simulink model "Sim_2025_04_07_Heet"  (R2024b)
settings: Solver=FixedStepAuto  StartTime=0.0  StopTime=2350  FixedStep=0.01  RelTol=1e-3
values from neighbouring files (symbols this model uses):
  cpSn = 230    [Sim_Parameter_Heet.m]
  mB = VB*rohSn    (= 7671.14496)    [Sim_Parameter_Heet.m]
  TU = 35    [Sim_Parameter_Heet.m]
undefined symbols (not defined in the file or in its folder): PLC_1, SIMATIC, UA
libraries: simulink x7, slpidlib x7, opcualib x6
(part 2 of 3)

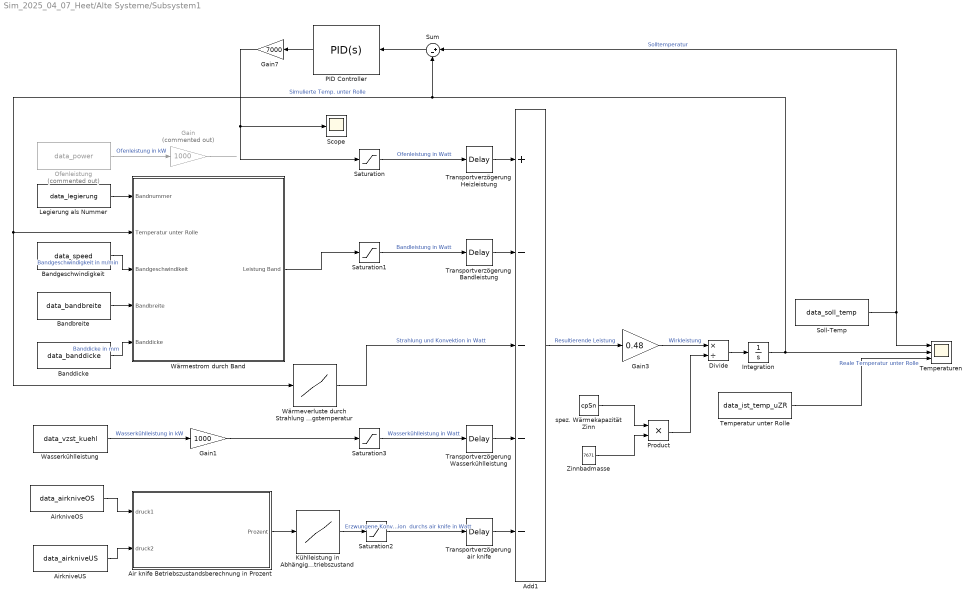
== system Sim_2025_04_07_Heet/Alte Systeme/Subsystem1 ==
  Add1 : Sum  Inputs=+----
  Air knife Betriebszustandsberechnung in Prozent : MATLAB Function  TreatAsAtomicUnit=on  SystemSampleTime=0.1
  AirkniveOS : FromWorkspace  VariableName=data_airkniveOS  SampleTime=-1
  AirkniveUS : FromWorkspace  VariableName=data_airkniveUS  SampleTime=-1
  Bandbreite : FromWorkspace  VariableName=data_bandbreite  SampleTime=-1
  Banddicke : FromWorkspace  VariableName=data_banddicke  SampleTime=-1
  Bandgeschwindigkeit : FromWorkspace  VariableName=data_speed  SampleTime=-1
  Divide : Product  Inputs=*/
  Gain : Gain  Commented=on  Gain=1000
  Gain1 : Gain  Gain=1000
  Gain3 : Gain  Gain=0.48
  Gain7 : Gain  Gain=7000
  Integration : Integrator  InitialCondition=264  IgnoreLimit=on
  Kühlleistung in Abhängigkeit des Betriebszustand : Lookup_n-D  NumberOfTableDimensions=1  BreakpointsForDimension1=[0 50 70 80 90 100]  Table=[0 25000 26500 26700 26900 26800]  InternalRulePriority=Speed  RndMeth=Simplest
  Legierung als Nummer : FromWorkspace  VariableName=data_legierung
  Ofenleistung : FromWorkspace  Commented=on  VariableName=data_power  SampleTime=-1  OutputAfterFinalValue=Setting to zero
  PID Controller : slpidlib/PID Controller  Controller=PID  Form=Parallel  TimeDomain=Continuous-time  UseExternalTs=off  SampleTime=-1  IntegratorMethod=Forward Euler  FilterMethod=Forward Euler  ControllerParametersSource=internal  P=5  I=0.015  UseKiTs=off  D=40  UseExternalDerivativeSource=off  N=1  UseFilter=on  TunerSelectOption=Transfer Function Based (PID Tuner App)  InitialConditionSource=internal  InitialConditionForIntegrator=0  InitialConditionForFilter=0  DifferentiatorICPrevScaledInput=0  ExternalReset=none  TrackingMode=off  Kt=1  LimitOutput=on  SatLimitsSource=internal  UpperSaturationLimit=100  LowerSaturationLimit=0  LinearizeAsGain=on  AntiWindupMode=back-calculation  Kb=1  LimitIntegrator=off  UpperIntegratorSaturationLimit=inf  LowerIntegratorSaturationLimit=-inf  POutMin=[]  POutMax=[]  IOutMin=[]  IOutMax=[]  DOutMin=[]  DOutMax=[]  NOutMin=[]  NOutMax=[]  SumOutMin=[]  SumOutMax=[]  SaturationOutMin=[]  SaturationOutMax=[]  PParamMin=[]  PParamMax=[]  IParamMin=[]  IParamMax=[]  DParamMin=[]  DParamMax=[]  NParamMin=[]  NParamMax=[]  KbParamMin=[]  KbParamMax=[]  KtParamMin=[]  KtParamMax=[]  KbOutMin=[]  KbOutMax=[]  KtOutMin=[]  KtOutMax=[]  IntegratorOutMin=[]  IntegratorOutMax=[]  FilterOutMin=[]  FilterOutMax=[]  SumI1OutMin=[]  SumI1OutMax=[]  SumI2OutMin=[]  SumI2OutMax=[]  SumI3OutMin=[]  SumI3OutMax=[]  SumI4OutMin=[]  SumI4OutMax=[]  SumDOutMin=[]  SumDOutMax=[]  DifferentiatorOutMin=[]  DifferentiatorOutMax=[]  FilterDiffOutCoefMin=[]  FilterDiffOutCoefMax=[]  ReciprocalOutMin=[]  ReciprocalOutMax=[]  SumDenOutMin=[]  SumDenOutMax=[]  SumNumOutMin=[]  SumNumOutMax=[]  DivideOutMin=[]  DivideOutMax=[]  UdiffTsProdOutMin=[]  UdiffTsProdOutMax=[]  NTsProdOutMin=[]  NTsProdOutMax=[]  UintegralTsProdOutMin=[]  UintegralTsProdOutMax=[]  UngainTsProdOutMin=[]  UngainTsProdOutMax=[]  ClampingZeroOutDataTypeStr=Inherit: Inherit via back propagation  ClampingZeroOutMin=[]  ClampingZeroOutMax=[]  FilterDenConstantOutDataTypeStr=Inherit: Inherit via back propagation  FilterDenConstantOutMin=[]  FilterDenConstantOutMax=[]  PCopyOutDataTypeStr=Inherit: Inherit via back propagation  PCopyOutMin=[]  PCopyOutMax=[]  NCopyOutDataTypeStr=Inherit: Inherit via back propagation  NCopyOutMin=[]  NCopyOutMax=[]  IntegratorContinuousStateAttributes=''  IntegratorStateMustResolveToSignalObject=off  IntegratorRTWStateStorageClass=Auto  FilterContinuousStateAttributes=''  FilterStateMustResolveToSignalObject=off  FilterRTWStateStorageClass=Auto  ParallelPVariant=InternalParameters  IdealPVariant=Disabled  IVariant=InternalParameters  DVariant=InternalParameters  IntegratorVariant=Continuous  SatVariant=Enabled  AWVariant=BackCalculation  PCopyVariant=Disabled  TRVariant=Disabled  FdbkBlocksVariant=Forward  IdealPFdbkVariant=Disabled  SatFdbkVariant=Disabled  DerivativeFilterVariant=ContFilter  NVariant=InternalParameters  NCopyVariant=Disabled  FilterICVariant=InternalICsFilter  IntegratorICVariant=InternalICs  ExternalResetVariant=Disabled  TRSumVariant=Passthrough  SumFdbkVariant=Disabled  SumVariant=Sum_PID  TsampFilterVariant=InternalTs  TsampNgainVariant=Passthrough  TsampIntegralVariant=Disabled_SignalSpec  ExternalSaturationOutDataTypeStr=Inherit: Same as second input  DerivativeSourceVariant=ErrorSignal  PreIntVariant=InternalPreInt
  Product : Product
  Saturation{,1..3} (4 alike) : Saturate  UpperLimit=inf  LowerLimit=0
  Scope : Scope
  Soll-Temp : FromWorkspace  VariableName=data_soll_temp  SampleTime=-1
  Sum : Sum  Inputs=|+-
  Temperatur unter Rolle : FromWorkspace  VariableName=data_ist_temp_uZR  SampleTime=-1  OutputAfterFinalValue=Setting to zero
  Temperaturen : Scope  NumInputPorts=3
  Transportverzögerung Bandleistung : TransportDelay  DelayTime=5
  Transportverzögerung Heizleistung : TransportDelay  DelayTime=94  BufferSize=15000
  Transportverzögerung Wasserkühlleistung : TransportDelay  DelayTime=94
  Transportverzögerung air knife : TransportDelay  DelayTime=0  BufferSize=20480
  Wasserkühlleistung : FromWorkspace  VariableName=data_vzst_kuehl  SampleTime=-1
  Wärmestrom durch Band : Subsystem
  "Wärmeverluste durch Strahlung und Konvektion in Abhängigkeit der Zinntemperatur, mit fester Umgebungstemperatur" : Lookup_n-D  NumberOfTableDimensions=1  BreakpointsForDimension1=[0 250 260 270 280 290 300 310 320]  Table=[0;20500;22000;23500;25000;27500;30000;33000;37000]  InternalRulePriority=Speed  RndMeth=Simplest
  Zinnbadmasse : Constant  Value=7671
  spez. Wärmekapazität Zinn : Constant  Value=cpSn
  wires:
  Gain/1 -> ?
  Ofenleistung/1 -> Gain/1  "Ofenleistung in kW"
  Wärmestrom durch Band/1(Leistung Band) -> Saturation1/1
  Temperatur unter Rolle/1 -> Temperaturen/3  "Reale Temperatur unter Rolle"
  Gain3/1 -> Divide/1  "Wirkleistung"
  Kühlleistung in Abhängigkeit des Betriebszustand/1 -> Saturation2/1
  "Wärmeverluste durch Strahlung und Konvektion in Abhängigkeit der Zinntemperatur, mit fester Umgebungstemperatur"/1 -> Add1/3  "Strahlung und Konvektion in Watt"
  Zinnbadmasse/1 -> Product/2
  AirkniveUS/1 -> Air knife Betriebszustandsberechnung in Prozent/2(druck2)
  Integration/1 -> "Wärmeverluste durch Strahlung und Konvektion in Abhängigkeit der Zinntemperatur, mit fester Umgebungstemperatur"/1, Wärmestrom durch Band/2(Temperatur unter Rolle), Sum/2, Temperaturen/2  "Simulierte Temp. unter Rolle"
  Sum/1 -> PID Controller/1
  Soll-Temp/1 -> Temperaturen/1, Sum/1  "Solltemperatur"
  Air knife Betriebszustandsberechnung in Prozent/1(Prozent) -> Kühlleistung in Abhängigkeit des Betriebszustand/1
  Gain7/1 -> Saturation/1, Scope/1
  Divide/1 -> Integration/1
  Gain1/1 -> Saturation3/1
  AirkniveOS/1 -> Air knife Betriebszustandsberechnung in Prozent/1(druck1)
  spez. Wärmekapazität Zinn/1 -> Product/1
  Bandgeschwindigkeit/1 -> Wärmestrom durch Band/3(Bandgeschwindikeit)  "Bandgeschwindigkeit in m/min"
  Saturation3/1 -> Transportverzögerung Wasserkühlleistung/1  "Wasserkühlleistung in Watt"
  Add1/1 -> Gain3/1  "Resultierende Leistung"
  Saturation/1 -> Transportverzögerung Heizleistung/1  "Ofenleistung in Watt"
  Legierung als Nummer/1 -> Wärmestrom durch Band/1(Bandnummer)
  Wasserkühlleistung/1 -> Gain1/1  "Wasserkühlleistung in kW"
  Banddicke/1 -> Wärmestrom durch Band/5(Banddicke)  "Banddicke in mm"
  Bandbreite/1 -> Wärmestrom durch Band/4(Bandbreite)
  Transportverzögerung Bandleistung/1 -> Add1/2
  Saturation2/1 -> Transportverzögerung air knife/1  "Erzwungene Konvektion  durchs air knife in Watt"
  Transportverzögerung air knife/1 -> Add1/5
  Transportverzögerung Heizleistung/1 -> Add1/1
  PID Controller/1 -> Gain7/1
  Saturation1/1 -> Transportverzögerung Bandleistung/1  "Bandleistung in Watt"
  Transportverzögerung Wasserkühlleistung/1 -> Add1/4
  Product/1 -> Divide/2

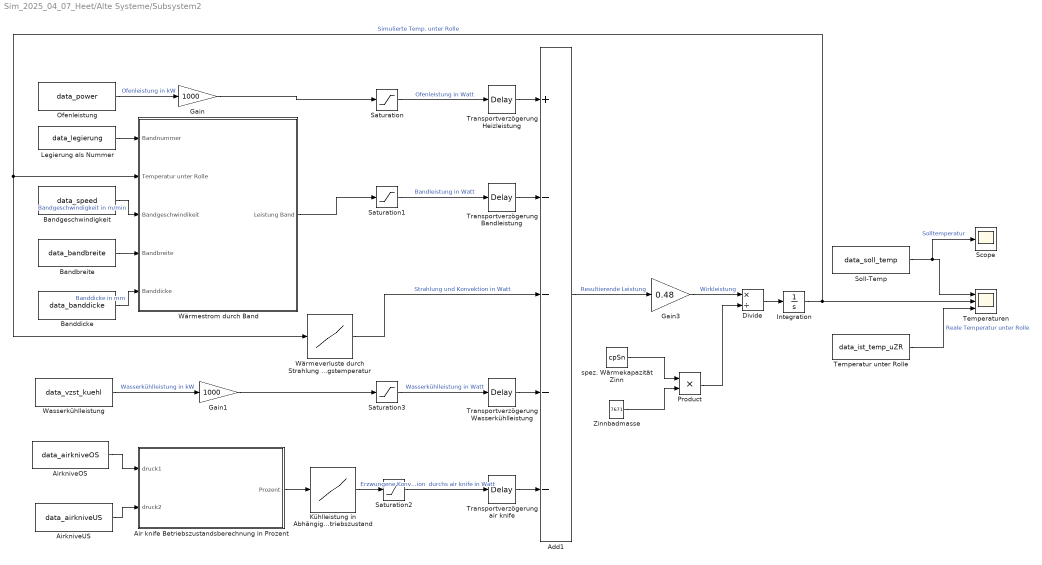
== system Sim_2025_04_07_Heet/Alte Systeme/Subsystem2 ==
  Add1 : Sum  Inputs=+----
  Air knife Betriebszustandsberechnung in Prozent : MATLAB Function  TreatAsAtomicUnit=on  SystemSampleTime=0.1
  AirkniveOS : FromWorkspace  VariableName=data_airkniveOS  SampleTime=-1
  AirkniveUS : FromWorkspace  VariableName=data_airkniveUS  SampleTime=-1
  Bandbreite : FromWorkspace  VariableName=data_bandbreite  SampleTime=-1
  Banddicke : FromWorkspace  VariableName=data_banddicke  SampleTime=-1
  Bandgeschwindigkeit : FromWorkspace  VariableName=data_speed  SampleTime=-1
  Divide : Product  Inputs=*/
  Gain : Gain  Gain=1000
  Gain1 : Gain  Gain=1000
  Gain3 : Gain  Gain=0.48
  Integration : Integrator  InitialCondition=264  IgnoreLimit=on
  Kühlleistung in Abhängigkeit des Betriebszustand : Lookup_n-D  NumberOfTableDimensions=1  BreakpointsForDimension1=[0 50 70 80 90 100]  Table=[0 25000 26500 26700 26900 26800]  InternalRulePriority=Speed  RndMeth=Simplest
  Legierung als Nummer : FromWorkspace  VariableName=data_legierung
  Ofenleistung : FromWorkspace  VariableName=data_power  SampleTime=-1  OutputAfterFinalValue=Setting to zero
  Product : Product
  Saturation{,1..3} (4 alike) : Saturate  UpperLimit=inf  LowerLimit=0
  Scope : Scope
  Soll-Temp : FromWorkspace  VariableName=data_soll_temp  SampleTime=-1
  Temperatur unter Rolle : FromWorkspace  VariableName=data_ist_temp_uZR  SampleTime=-1  OutputAfterFinalValue=Setting to zero
  Temperaturen : Scope  NumInputPorts=3
  Transportverzögerung Bandleistung : TransportDelay  DelayTime=5
  Transportverzögerung Heizleistung : TransportDelay  DelayTime=94  BufferSize=15000
  Transportverzögerung Wasserkühlleistung : TransportDelay  DelayTime=94
  Transportverzögerung air knife : TransportDelay  DelayTime=0  BufferSize=20480
  Wasserkühlleistung : FromWorkspace  VariableName=data_vzst_kuehl  SampleTime=-1
  Wärmestrom durch Band : Subsystem
  "Wärmeverluste durch Strahlung und Konvektion in Abhängigkeit der Zinntemperatur, mit fester Umgebungstemperatur" : Lookup_n-D  NumberOfTableDimensions=1  BreakpointsForDimension1=[0 250 260 270 280 290 300 310 320]  Table=[0;20500;22000;23500;25000;27500;30000;33000;37000]  InternalRulePriority=Speed  RndMeth=Simplest
  Zinnbadmasse : Constant  Value=7671
  spez. Wärmekapazität Zinn : Constant  Value=cpSn
  wires:
  Gain/1 -> Saturation/1
  Ofenleistung/1 -> Gain/1  "Ofenleistung in kW"
  Wärmestrom durch Band/1(Leistung Band) -> Saturation1/1
  Temperatur unter Rolle/1 -> Temperaturen/3  "Reale Temperatur unter Rolle"
  Gain3/1 -> Divide/1  "Wirkleistung"
  Kühlleistung in Abhängigkeit des Betriebszustand/1 -> Saturation2/1
  "Wärmeverluste durch Strahlung und Konvektion in Abhängigkeit der Zinntemperatur, mit fester Umgebungstemperatur"/1 -> Add1/3  "Strahlung und Konvektion in Watt"
  Zinnbadmasse/1 -> Product/2
  AirkniveUS/1 -> Air knife Betriebszustandsberechnung in Prozent/2(druck2)
  Integration/1 -> "Wärmeverluste durch Strahlung und Konvektion in Abhängigkeit der Zinntemperatur, mit fester Umgebungstemperatur"/1, Wärmestrom durch Band/2(Temperatur unter Rolle), Temperaturen/2  "Simulierte Temp. unter Rolle"
  Soll-Temp/1 -> Temperaturen/1, Scope/1  "Solltemperatur"
  Air knife Betriebszustandsberechnung in Prozent/1(Prozent) -> Kühlleistung in Abhängigkeit des Betriebszustand/1
  Divide/1 -> Integration/1
  Gain1/1 -> Saturation3/1
  AirkniveOS/1 -> Air knife Betriebszustandsberechnung in Prozent/1(druck1)
  spez. Wärmekapazität Zinn/1 -> Product/1
  Bandgeschwindigkeit/1 -> Wärmestrom durch Band/3(Bandgeschwindikeit)  "Bandgeschwindigkeit in m/min"
  Saturation3/1 -> Transportverzögerung Wasserkühlleistung/1  "Wasserkühlleistung in Watt"
  Add1/1 -> Gain3/1  "Resultierende Leistung"
  Saturation/1 -> Transportverzögerung Heizleistung/1  "Ofenleistung in Watt"
  Legierung als Nummer/1 -> Wärmestrom durch Band/1(Bandnummer)
  Wasserkühlleistung/1 -> Gain1/1  "Wasserkühlleistung in kW"
  Banddicke/1 -> Wärmestrom durch Band/5(Banddicke)  "Banddicke in mm"
  Bandbreite/1 -> Wärmestrom durch Band/4(Bandbreite)
  Transportverzögerung Bandleistung/1 -> Add1/2
  Saturation2/1 -> Transportverzögerung air knife/1  "Erzwungene Konvektion  durchs air knife in Watt"
  Transportverzögerung air knife/1 -> Add1/5
  Transportverzögerung Heizleistung/1 -> Add1/1
  Saturation1/1 -> Transportverzögerung Bandleistung/1  "Bandleistung in Watt"
  Transportverzögerung Wasserkühlleistung/1 -> Add1/4
  Product/1 -> Divide/2

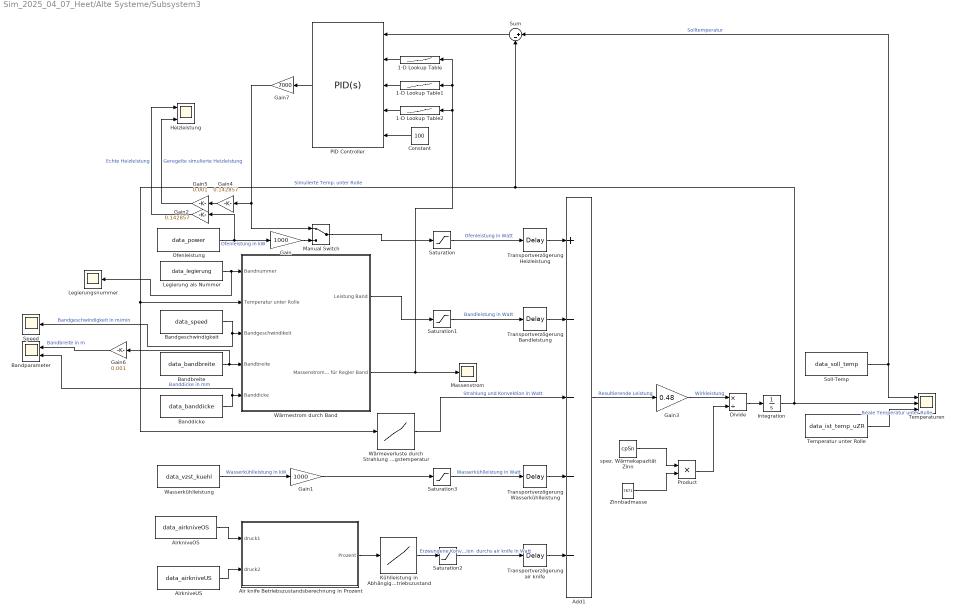
== system Sim_2025_04_07_Heet/Alte Systeme/Subsystem3 ==
  1-D Lookup Table : Lookup_n-D  NumberOfTableDimensions=1  BreakpointsForDimension1=[0 1.2]  Table=[5 6]  InternalRulePriority=Speed  RndMeth=Simplest
  1-D Lookup Table1 : Lookup_n-D  NumberOfTableDimensions=1  BreakpointsForDimension1=[0 1.2]  Table=[0.02 0.02]  InternalRulePriority=Speed  RndMeth=Simplest
  1-D Lookup Table2 : Lookup_n-D  NumberOfTableDimensions=1  BreakpointsForDimension1=[0 1.2]  Table=[0 30]  InternalRulePriority=Speed  RndMeth=Simplest
  Add1 : Sum  Inputs=+----
  Air knife Betriebszustandsberechnung in Prozent : MATLAB Function  TreatAsAtomicUnit=on  SystemSampleTime=0.1
  AirkniveOS : FromWorkspace  VariableName=data_airkniveOS  SampleTime=-1
  AirkniveUS : FromWorkspace  VariableName=data_airkniveUS  SampleTime=-1
  Bandbreite : FromWorkspace  VariableName=data_bandbreite  SampleTime=-1
  Banddicke : FromWorkspace  VariableName=data_banddicke  SampleTime=-1
  Bandgeschwindigkeit : FromWorkspace  VariableName=data_speed  SampleTime=-1
  Bandparameter : Scope  NumInputPorts=2
  Constant : Constant  Value=100
  Divide : Product  Inputs=*/
  Gain : Gain  Gain=1000
  Gain1 : Gain  Gain=1000
  Gain2 : Gain  Gain=0.142857
  Gain3 : Gain  Gain=0.48
  Gain4 : Gain  Gain=0.142857
  Gain5 : Gain  Gain=0.001
  Gain6 : Gain  Gain=0.001
  Gain7 : Gain  Gain=7000
  Heizleistung : Scope  NumInputPorts=2
  Integration : Integrator  InitialCondition=264  IgnoreLimit=on
  Kühlleistung in Abhängigkeit des Betriebszustand : Lookup_n-D  NumberOfTableDimensions=1  BreakpointsForDimension1=[0 50 70 80 90 100]  Table=[0 25000 26500 26700 26900 26800]  InternalRulePriority=Speed  RndMeth=Simplest
  Legierung als Nummer : FromWorkspace  VariableName=data_legierung
  Legierungsnummer : Scope
  Manual Switch : ManualSwitch
  Massenstrom : Scope
  Ofenleistung : FromWorkspace  VariableName=data_power  SampleTime=-1  OutputAfterFinalValue=Setting to zero
  PID Controller : slpidlib/PID Controller  Controller=PID  Form=Parallel  TimeDomain=Continuous-time  UseExternalTs=off  SampleTime=-1  IntegratorMethod=Forward Euler  FilterMethod=Forward Euler  ControllerParametersSource=external  P=5  I=0.015  UseKiTs=off  D=40  UseExternalDerivativeSource=off  N=1  UseFilter=on  TunerSelectOption=Transfer Function Based (PID Tuner App)  InitialConditionSource=internal  InitialConditionForIntegrator=0  InitialConditionForFilter=0  DifferentiatorICPrevScaledInput=0  ExternalReset=none  TrackingMode=off  Kt=1  LimitOutput=on  SatLimitsSource=internal  UpperSaturationLimit=100  LowerSaturationLimit=0  LinearizeAsGain=on  AntiWindupMode=back-calculation  Kb=1  LimitIntegrator=off  UpperIntegratorSaturationLimit=inf  LowerIntegratorSaturationLimit=-inf  POutMin=[]  POutMax=[]  IOutMin=[]  IOutMax=[]  DOutMin=[]  DOutMax=[]  NOutMin=[]  NOutMax=[]  SumOutMin=[]  SumOutMax=[]  SaturationOutMin=[]  SaturationOutMax=[]  PParamMin=[]  PParamMax=[]  IParamMin=[]  IParamMax=[]  DParamMin=[]  DParamMax=[]  NParamMin=[]  NParamMax=[]  KbParamMin=[]  KbParamMax=[]  KtParamMin=[]  KtParamMax=[]  KbOutMin=[]  KbOutMax=[]  KtOutMin=[]  KtOutMax=[]  IntegratorOutMin=[]  IntegratorOutMax=[]  FilterOutMin=[]  FilterOutMax=[]  SumI1OutMin=[]  SumI1OutMax=[]  SumI2OutMin=[]  SumI2OutMax=[]  SumI3OutMin=[]  SumI3OutMax=[]  SumI4OutMin=[]  SumI4OutMax=[]  SumDOutMin=[]  SumDOutMax=[]  DifferentiatorOutMin=[]  DifferentiatorOutMax=[]  FilterDiffOutCoefMin=[]  FilterDiffOutCoefMax=[]  ReciprocalOutMin=[]  ReciprocalOutMax=[]  SumDenOutMin=[]  SumDenOutMax=[]  SumNumOutMin=[]  SumNumOutMax=[]  DivideOutMin=[]  DivideOutMax=[]  UdiffTsProdOutMin=[]  UdiffTsProdOutMax=[]  NTsProdOutMin=[]  NTsProdOutMax=[]  UintegralTsProdOutMin=[]  UintegralTsProdOutMax=[]  UngainTsProdOutMin=[]  UngainTsProdOutMax=[]  ClampingZeroOutDataTypeStr=Inherit: Inherit via back propagation  ClampingZeroOutMin=[]  ClampingZeroOutMax=[]  FilterDenConstantOutDataTypeStr=Inherit: Inherit via back propagation  FilterDenConstantOutMin=[]  FilterDenConstantOutMax=[]  PCopyOutDataTypeStr=Inherit: Inherit via back propagation  PCopyOutMin=[]  PCopyOutMax=[]  NCopyOutDataTypeStr=Inherit: Inherit via back propagation  NCopyOutMin=[]  NCopyOutMax=[]  IntegratorContinuousStateAttributes=''  IntegratorStateMustResolveToSignalObject=off  IntegratorRTWStateStorageClass=Auto  FilterContinuousStateAttributes=''  FilterStateMustResolveToSignalObject=off  FilterRTWStateStorageClass=Auto  ParallelPVariant=ExternalParameters  IdealPVariant=Disabled  IVariant=ExternalParameters  DVariant=ExternalParameters  IntegratorVariant=Continuous  SatVariant=Enabled  AWVariant=BackCalculation  PCopyVariant=Disabled  TRVariant=Disabled  FdbkBlocksVariant=Forward  IdealPFdbkVariant=Disabled  SatFdbkVariant=Disabled  DerivativeFilterVariant=ContFilter  NVariant=ExternalParameters  NCopyVariant=Disabled  FilterICVariant=InternalICsFilter  IntegratorICVariant=InternalICs  ExternalResetVariant=Disabled  TRSumVariant=Passthrough  SumFdbkVariant=Disabled  SumVariant=Sum_PID  TsampFilterVariant=InternalTs  TsampNgainVariant=Passthrough  TsampIntegralVariant=Disabled_SignalSpec  ExternalSaturationOutDataTypeStr=Inherit: Same as second input  DerivativeSourceVariant=ErrorSignal  PreIntVariant=InternalPreInt
  Product : Product
  Saturation{,1..3} (4 alike) : Saturate  UpperLimit=inf  LowerLimit=0
  Soll-Temp : FromWorkspace  VariableName=data_soll_temp  SampleTime=-1
  Speed : Scope
  Sum : Sum  Inputs=|+-
  Temperatur unter Rolle : FromWorkspace  VariableName=data_ist_temp_uZR  SampleTime=-1  OutputAfterFinalValue=Setting to zero
  Temperaturen : Scope  NumInputPorts=3
  Transportverzögerung Bandleistung : TransportDelay  DelayTime=5
  Transportverzögerung Heizleistung : TransportDelay  DelayTime=94  BufferSize=15000
  Transportverzögerung Wasserkühlleistung : TransportDelay  DelayTime=94
  Transportverzögerung air knife : TransportDelay  DelayTime=0  BufferSize=20480
  Wasserkühlleistung : FromWorkspace  VariableName=data_vzst_kuehl  SampleTime=-1
  Wärmestrom durch Band : Subsystem
  "Wärmeverluste durch Strahlung und Konvektion in Abhängigkeit der Zinntemperatur, mit fester Umgebungstemperatur" : Lookup_n-D  NumberOfTableDimensions=1  BreakpointsForDimension1=[0 250 260 270 280 290 300 310 320]  Table=[0;20500;22000;23500;25000;27500;30000;33000;37000]  InternalRulePriority=Speed  RndMeth=Simplest
  Zinnbadmasse : Constant  Value=7671
  spez. Wärmekapazität Zinn : Constant  Value=cpSn
  wires:
  Gain6/1 -> Bandparameter/1  "Bandbreite in m"
  Wärmestrom durch Band/2(Massenstrom für Regler Band) -> 1-D Lookup Table/1, 1-D Lookup Table1/1, 1-D Lookup Table2/1, Massenstrom/1
  Constant/1 -> PID Controller/5
  1-D Lookup Table2/1 -> PID Controller/4
  1-D Lookup Table1/1 -> PID Controller/3
  1-D Lookup Table/1 -> PID Controller/2
  Wärmestrom durch Band/1(Leistung Band) -> Saturation1/1
  Temperatur unter Rolle/1 -> Temperaturen/3  "Reale Temperatur unter Rolle"
  Gain3/1 -> Divide/1  "Wirkleistung"
  Kühlleistung in Abhängigkeit des Betriebszustand/1 -> Saturation2/1
  "Wärmeverluste durch Strahlung und Konvektion in Abhängigkeit der Zinntemperatur, mit fester Umgebungstemperatur"/1 -> Add1/3  "Strahlung und Konvektion in Watt"
  Ofenleistung/1 -> Gain2/1, Gain/1  "Ofenleistung in kW"
  Zinnbadmasse/1 -> Product/2
  AirkniveUS/1 -> Air knife Betriebszustandsberechnung in Prozent/2(druck2)
  Integration/1 -> "Wärmeverluste durch Strahlung und Konvektion in Abhängigkeit der Zinntemperatur, mit fester Umgebungstemperatur"/1, Wärmestrom durch Band/2(Temperatur unter Rolle), Sum/2, Temperaturen/2  "Simulierte Temp. unter Rolle"
  Gain7/1 -> Gain4/1, Manual Switch/1
  Sum/1 -> PID Controller/1
  Gain5/1 -> Heizleistung/2  "Geregelte simulierte Heizleistung"
  Soll-Temp/1 -> Temperaturen/1, Sum/1  "Solltemperatur"
  Air knife Betriebszustandsberechnung in Prozent/1(Prozent) -> Kühlleistung in Abhängigkeit des Betriebszustand/1
  Manual Switch/1 -> Saturation/1
  Divide/1 -> Integration/1
  Gain1/1 -> Saturation3/1
  AirkniveOS/1 -> Air knife Betriebszustandsberechnung in Prozent/1(druck1)
  spez. Wärmekapazität Zinn/1 -> Product/1
  Gain4/1 -> Gain5/1
  Gain/1 -> Manual Switch/2
  Bandgeschwindigkeit/1 -> Wärmestrom durch Band/3(Bandgeschwindikeit), Speed/1  "Bandgeschwindigkeit in m/min"
  Saturation3/1 -> Transportverzögerung Wasserkühlleistung/1  "Wasserkühlleistung in Watt"
  Add1/1 -> Gain3/1  "Resultierende Leistung"
  Gain2/1 -> Heizleistung/1  "Echte Heizleistung"
  Saturation/1 -> Transportverzögerung Heizleistung/1  "Ofenleistung in Watt"
  Legierung als Nummer/1 -> Legierungsnummer/1, Wärmestrom durch Band/1(Bandnummer)
  Wasserkühlleistung/1 -> Gain1/1  "Wasserkühlleistung in kW"
  Banddicke/1 -> Wärmestrom durch Band/5(Banddicke), Bandparameter/2  "Banddicke in mm"
  Bandbreite/1 -> Wärmestrom durch Band/4(Bandbreite), Gain6/1
  Transportverzögerung Bandleistung/1 -> Add1/2
  Saturation2/1 -> Transportverzögerung air knife/1  "Erzwungene Konvektion  durchs air knife in Watt"
  Transportverzögerung air knife/1 -> Add1/5
  Transportverzögerung Heizleistung/1 -> Add1/1
  PID Controller/1 -> Gain7/1
  Saturation1/1 -> Transportverzögerung Bandleistung/1  "Bandleistung in Watt"
  Transportverzögerung Wasserkühlleistung/1 -> Add1/4
  Product/1 -> Divide/2

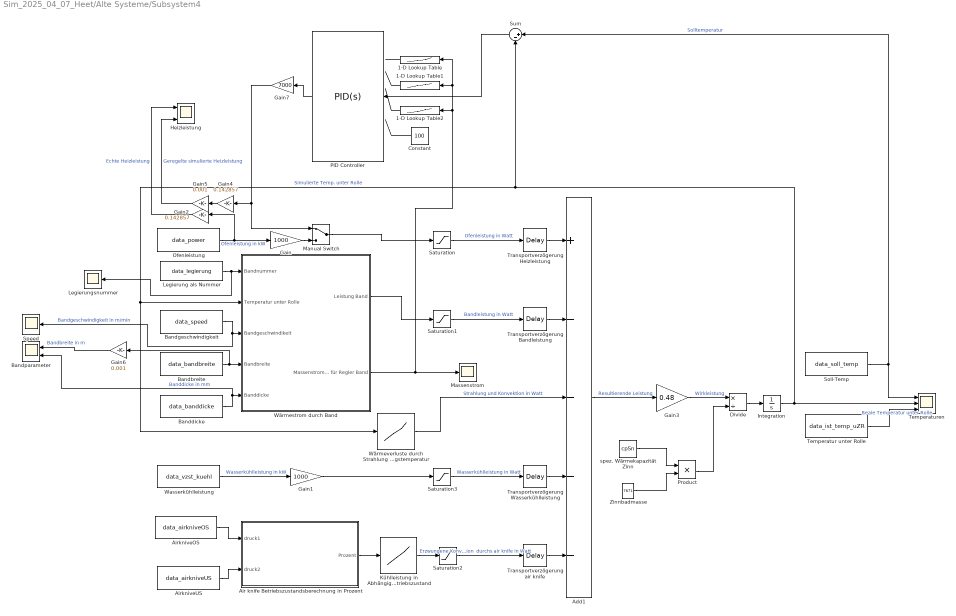
== system Sim_2025_04_07_Heet/Alte Systeme/Subsystem4 ==
  1-D Lookup Table : Lookup_n-D  NumberOfTableDimensions=1  BreakpointsForDimension1=[0 0.29999999999999999 0.59999999999999998 0.90000000000000002 1.2 1.5 1.8 2.1000000000000001 2.3999999999999999 2.7000000000000002 3 3.2999999999999998 3.6000000000000001 3.8999999999999999 4.2000000000000002 4.5]  Table=[4;4.2;4.4;4.6;4.8;5;5.2;5.4;5.6;5.8;6;6.2;6.4;6.6;6.8;7]  InternalRulePriority=Speed  RndMeth=Simplest
  1-D Lookup Table1 : Lookup_n-D  NumberOfTableDimensions=1  BreakpointsForDimension1=[0 0.29999999999999999 0.59999999999999998 0.90000000000000002 1.2 1.5 1.8 2.1000000000000001 2.3999999999999999 2.7000000000000002 3 3.2999999999999998 3.6000000000000001 3.8999999999999999 4.2000000000000002 4.5]  Table=[0.02;0.02;0.02;0.02;0.02;0.02;0.02;0.02;0.02;0.02;0.02;0.02;0.02;0.02;0.02;0.02]  InternalRulePriority=Speed  RndMeth=Simplest
  1-D Lookup Table2 : Lookup_n-D  NumberOfTableDimensions=1  BreakpointsForDimension1=[0 0.29999999999999999 0.59999999999999998 0.90000000000000002 1.2 1.5 1.8 2.1000000000000001 2.3999999999999999 2.7000000000000002 3 3.2999999999999998 3.6000000000000001 3.8999999999999999 4.2000000000000002 4.5]  Table=[30;30;30;30;30;30;30;30;30;30;30;30;30;30;30;30]  InternalRulePriority=Speed  RndMeth=Simplest
  Add1 : Sum  Inputs=+----
  Air knife Betriebszustandsberechnung in Prozent : MATLAB Function  TreatAsAtomicUnit=on  SystemSampleTime=0.1
  AirkniveOS : FromWorkspace  VariableName=data_airkniveOS  SampleTime=-1
  AirkniveUS : FromWorkspace  VariableName=data_airkniveUS  SampleTime=-1
  Bandbreite : FromWorkspace  VariableName=data_bandbreite  SampleTime=-1
  Banddicke : FromWorkspace  VariableName=data_banddicke  SampleTime=-1
  Bandgeschwindigkeit : FromWorkspace  VariableName=data_speed  SampleTime=-1
  Bandparameter : Scope  NumInputPorts=2
  Constant : Constant  Value=100
  Divide : Product  Inputs=*/
  Gain : Gain  Gain=1000
  Gain1 : Gain  Gain=1000
  Gain2 : Gain  Gain=0.142857
  Gain3 : Gain  Gain=0.48
  Gain4 : Gain  Gain=0.142857
  Gain5 : Gain  Gain=0.001
  Gain6 : Gain  Gain=0.001
  Gain7 : Gain  Gain=7000
  Heizleistung : Scope  NumInputPorts=2
  Integration : Integrator  InitialCondition=273  IgnoreLimit=on
  Kühlleistung in Abhängigkeit des Betriebszustand : Lookup_n-D  NumberOfTableDimensions=1  BreakpointsForDimension1=[0 50 70 80 90 100]  Table=[0 25000 26500 26700 26900 26800]  InternalRulePriority=Speed  RndMeth=Simplest
  Legierung als Nummer : FromWorkspace  VariableName=data_legierung
  Legierungsnummer : Scope
  Manual Switch : ManualSwitch
  Massenstrom : Scope
  Ofenleistung : FromWorkspace  VariableName=data_power  SampleTime=-1  OutputAfterFinalValue=Setting to zero
  PID Controller : slpidlib/PID Controller  Controller=PID  Form=Parallel  TimeDomain=Continuous-time  UseExternalTs=off  SampleTime=-1  IntegratorMethod=Forward Euler  FilterMethod=Forward Euler  ControllerParametersSource=internal  P=5  I=0.012  UseKiTs=off  D=5  UseExternalDerivativeSource=off  N=1  UseFilter=on  TunerSelectOption=Transfer Function Based (PID Tuner App)  InitialConditionSource=internal  InitialConditionForIntegrator=0  InitialConditionForFilter=0  DifferentiatorICPrevScaledInput=0  ExternalReset=none  TrackingMode=off  Kt=1  LimitOutput=on  SatLimitsSource=internal  UpperSaturationLimit=100  LowerSaturationLimit=0  LinearizeAsGain=on  AntiWindupMode=back-calculation  Kb=1  LimitIntegrator=off  UpperIntegratorSaturationLimit=inf  LowerIntegratorSaturationLimit=-inf  POutMin=[]  POutMax=[]  IOutMin=[]  IOutMax=[]  DOutMin=[]  DOutMax=[]  NOutMin=[]  NOutMax=[]  SumOutMin=[]  SumOutMax=[]  SaturationOutMin=[]  SaturationOutMax=[]  PParamMin=[]  PParamMax=[]  IParamMin=[]  IParamMax=[]  DParamMin=[]  DParamMax=[]  NParamMin=[]  NParamMax=[]  KbParamMin=[]  KbParamMax=[]  KtParamMin=[]  KtParamMax=[]  KbOutMin=[]  KbOutMax=[]  KtOutMin=[]  KtOutMax=[]  IntegratorOutMin=[]  IntegratorOutMax=[]  FilterOutMin=[]  FilterOutMax=[]  SumI1OutMin=[]  SumI1OutMax=[]  SumI2OutMin=[]  SumI2OutMax=[]  SumI3OutMin=[]  SumI3OutMax=[]  SumI4OutMin=[]  SumI4OutMax=[]  SumDOutMin=[]  SumDOutMax=[]  DifferentiatorOutMin=[]  DifferentiatorOutMax=[]  FilterDiffOutCoefMin=[]  FilterDiffOutCoefMax=[]  ReciprocalOutMin=[]  ReciprocalOutMax=[]  SumDenOutMin=[]  SumDenOutMax=[]  SumNumOutMin=[]  SumNumOutMax=[]  DivideOutMin=[]  DivideOutMax=[]  UdiffTsProdOutMin=[]  UdiffTsProdOutMax=[]  NTsProdOutMin=[]  NTsProdOutMax=[]  UintegralTsProdOutMin=[]  UintegralTsProdOutMax=[]  UngainTsProdOutMin=[]  UngainTsProdOutMax=[]  ClampingZeroOutDataTypeStr=Inherit: Inherit via back propagation  ClampingZeroOutMin=[]  ClampingZeroOutMax=[]  FilterDenConstantOutDataTypeStr=Inherit: Inherit via back propagation  FilterDenConstantOutMin=[]  FilterDenConstantOutMax=[]  PCopyOutDataTypeStr=Inherit: Inherit via back propagation  PCopyOutMin=[]  PCopyOutMax=[]  NCopyOutDataTypeStr=Inherit: Inherit via back propagation  NCopyOutMin=[]  NCopyOutMax=[]  IntegratorContinuousStateAttributes=''  IntegratorStateMustResolveToSignalObject=off  IntegratorRTWStateStorageClass=Auto  FilterContinuousStateAttributes=''  FilterStateMustResolveToSignalObject=off  FilterRTWStateStorageClass=Auto  ParallelPVariant=InternalParameters  IdealPVariant=Disabled  IVariant=InternalParameters  DVariant=InternalParameters  IntegratorVariant=Continuous  SatVariant=Enabled  AWVariant=BackCalculation  PCopyVariant=Disabled  TRVariant=Disabled  FdbkBlocksVariant=Forward  IdealPFdbkVariant=Disabled  SatFdbkVariant=Disabled  DerivativeFilterVariant=ContFilter  NVariant=InternalParameters  NCopyVariant=Disabled  FilterICVariant=InternalICsFilter  IntegratorICVariant=InternalICs  ExternalResetVariant=Disabled  TRSumVariant=Passthrough  SumFdbkVariant=Disabled  SumVariant=Sum_PID  TsampFilterVariant=InternalTs  TsampNgainVariant=Passthrough  TsampIntegralVariant=Disabled_SignalSpec  ExternalSaturationOutDataTypeStr=Inherit: Same as second input  DerivativeSourceVariant=ErrorSignal  PreIntVariant=InternalPreInt
  Product : Product
  Saturation{,1..3} (4 alike) : Saturate  UpperLimit=inf  LowerLimit=0
  Soll-Temp : FromWorkspace  VariableName=data_soll_temp  SampleTime=-1
  Speed : Scope
  Sum : Sum  Inputs=|+-
  Temperatur unter Rolle : FromWorkspace  VariableName=data_ist_temp_uZR  SampleTime=-1  OutputAfterFinalValue=Setting to zero
  Temperaturen : Scope  NumInputPorts=3
  Transportverzögerung Bandleistung : TransportDelay  DelayTime=5
  Transportverzögerung Heizleistung : TransportDelay  DelayTime=94  BufferSize=15000
  Transportverzögerung Wasserkühlleistung : TransportDelay  DelayTime=94
  Transportverzögerung air knife : TransportDelay  DelayTime=0  BufferSize=20480
  Wasserkühlleistung : FromWorkspace  VariableName=data_vzst_kuehl  SampleTime=-1
  Wärmestrom durch Band : Subsystem
  "Wärmeverluste durch Strahlung und Konvektion in Abhängigkeit der Zinntemperatur, mit fester Umgebungstemperatur" : Lookup_n-D  NumberOfTableDimensions=1  BreakpointsForDimension1=[0 250 260 270 280 290 300 310 320]  Table=[0;20500;22000;23500;25000;27500;30000;33000;37000]  InternalRulePriority=Speed  RndMeth=Simplest
  Zinnbadmasse : Constant  Value=7671
  spez. Wärmekapazität Zinn : Constant  Value=cpSn
  wires:
  Gain6/1 -> Bandparameter/1  "Bandbreite in m"
  Wärmestrom durch Band/2(Massenstrom für Regler Band) -> 1-D Lookup Table/1, 1-D Lookup Table1/1, 1-D Lookup Table2/1, Massenstrom/1
  Constant/1 -> ?
  1-D Lookup Table2/1 -> ?
  1-D Lookup Table1/1 -> ?
  1-D Lookup Table/1 -> ?
  Wärmestrom durch Band/1(Leistung Band) -> Saturation1/1
  Temperatur unter Rolle/1 -> Temperaturen/3  "Reale Temperatur unter Rolle"
  Gain3/1 -> Divide/1  "Wirkleistung"
  Kühlleistung in Abhängigkeit des Betriebszustand/1 -> Saturation2/1
  "Wärmeverluste durch Strahlung und Konvektion in Abhängigkeit der Zinntemperatur, mit fester Umgebungstemperatur"/1 -> Add1/3  "Strahlung und Konvektion in Watt"
  Ofenleistung/1 -> Gain2/1, Gain/1  "Ofenleistung in kW"
  Zinnbadmasse/1 -> Product/2
  AirkniveUS/1 -> Air knife Betriebszustandsberechnung in Prozent/2(druck2)
  Integration/1 -> "Wärmeverluste durch Strahlung und Konvektion in Abhängigkeit der Zinntemperatur, mit fester Umgebungstemperatur"/1, Wärmestrom durch Band/2(Temperatur unter Rolle), Sum/2, Temperaturen/2  "Simulierte Temp. unter Rolle"
  Gain7/1 -> Gain4/1, Manual Switch/1
  Sum/1 -> PID Controller/1
  Gain5/1 -> Heizleistung/2  "Geregelte simulierte Heizleistung"
  Soll-Temp/1 -> Temperaturen/1, Sum/1  "Solltemperatur"
  Air knife Betriebszustandsberechnung in Prozent/1(Prozent) -> Kühlleistung in Abhängigkeit des Betriebszustand/1
  Manual Switch/1 -> Saturation/1
  Divide/1 -> Integration/1
  Gain1/1 -> Saturation3/1
  AirkniveOS/1 -> Air knife Betriebszustandsberechnung in Prozent/1(druck1)
  spez. Wärmekapazität Zinn/1 -> Product/1
  Gain4/1 -> Gain5/1
  Gain/1 -> Manual Switch/2
  Bandgeschwindigkeit/1 -> Wärmestrom durch Band/3(Bandgeschwindikeit), Speed/1  "Bandgeschwindigkeit in m/min"
  Saturation3/1 -> Transportverzögerung Wasserkühlleistung/1  "Wasserkühlleistung in Watt"
  Add1/1 -> Gain3/1  "Resultierende Leistung"
  Gain2/1 -> Heizleistung/1  "Echte Heizleistung"
  Saturation/1 -> Transportverzögerung Heizleistung/1  "Ofenleistung in Watt"
  Legierung als Nummer/1 -> Legierungsnummer/1, Wärmestrom durch Band/1(Bandnummer)
  Wasserkühlleistung/1 -> Gain1/1  "Wasserkühlleistung in kW"
  Banddicke/1 -> Wärmestrom durch Band/5(Banddicke), Bandparameter/2  "Banddicke in mm"
  Bandbreite/1 -> Wärmestrom durch Band/4(Bandbreite), Gain6/1
  Transportverzögerung Bandleistung/1 -> Add1/2
  Saturation2/1 -> Transportverzögerung air knife/1  "Erzwungene Konvektion  durchs air knife in Watt"
  Transportverzögerung air knife/1 -> Add1/5
  Transportverzögerung Heizleistung/1 -> Add1/1
  PID Controller/1 -> Gain7/1
  Saturation1/1 -> Transportverzögerung Bandleistung/1  "Bandleistung in Watt"
  Transportverzögerung Wasserkühlleistung/1 -> Add1/4
  Product/1 -> Divide/2

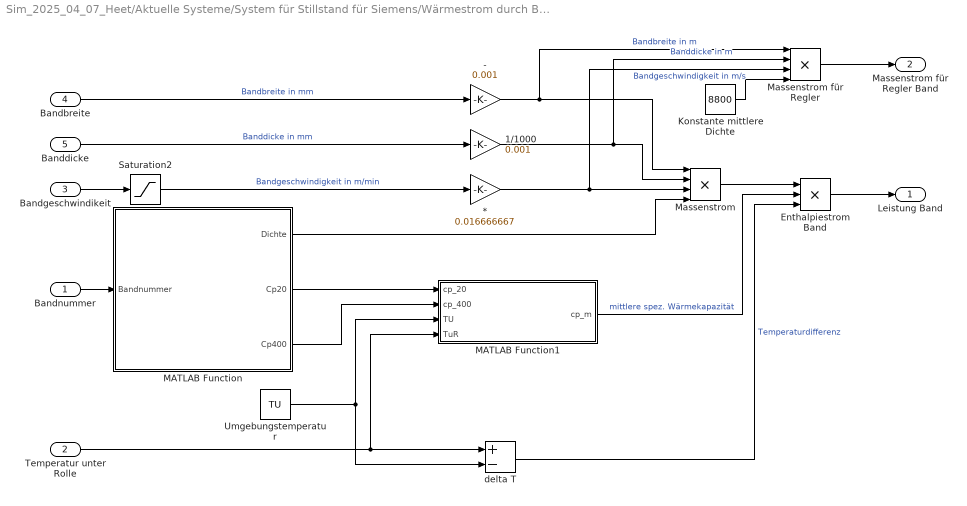
== system Sim_2025_04_07_Heet/Aktuelle Systeme/System für Stillstand für Siemens/Wärmestrom durch Band ==
  Bandnummer : Inport
  Temperatur unter Rolle : Inport  Port=2
  Bandgeschwindikeit : Inport  Port=3
  Bandbreite : Inport  Port=4
  Banddicke : Inport  Port=5
  * : Gain  Gain=0.016666667
  - : Gain  Gain=0.001
  1/1000 : Gain  Gain=0.001
  Enthalpiestrom Band : Product  Inputs=3
  Konstante mittlere Dichte : Constant  Value=8800
  MATLAB Function : MATLAB Function  TreatAsAtomicUnit=on
  MATLAB Function1 : MATLAB Function  TreatAsAtomicUnit=on
  Massenstrom : Product  Inputs=4
  Massenstrom für Regler : Product  Inputs=4
  Saturation2 : Saturate  UpperLimit=inf  LowerLimit=0
  Umgebungstemperatur : Constant  Value=TU
  delta T : Sum  Inputs=+-
  Leistung Band : Outport
  Massenstrom für Regler Band : Outport  Port=2
  wires:
  1/1000/1 -> Massenstrom für Regler/2, Massenstrom/2  "Banddicke in m"
  Temperatur unter Rolle/1 -> delta T/1, MATLAB Function1/4(TuR)
  Bandgeschwindikeit/1 -> Saturation2/1
  Banddicke/1 -> 1/1000/1  "Banddicke in mm"
  -/1 -> Massenstrom für Regler/1, Massenstrom/1  "Bandbreite in m"
  */1 -> Massenstrom für Regler/3, Massenstrom/3  "Bandgeschwindigkeit in m/s"
  Bandnummer/1 -> MATLAB Function/1(Bandnummer)
  MATLAB Function/1(Dichte) -> Massenstrom/4
  MATLAB Function1/1(cp_m) -> Enthalpiestrom Band/2  "mittlere spez. Wärmekapazität"
  Umgebungstemperatur/1 -> MATLAB Function1/3(TU), delta T/2
  MATLAB Function/3(Cp400) -> MATLAB Function1/2(cp_400)
  MATLAB Function/2(Cp20) -> MATLAB Function1/1(cp_20)
  delta T/1 -> Enthalpiestrom Band/3  "Temperaturdifferenz"
  Saturation2/1 -> */1  "Bandgeschwindigkeit in m/min"
  Enthalpiestrom Band/1 -> Leistung Band/1
  Massenstrom/1 -> Enthalpiestrom Band/1
  Bandbreite/1 -> -/1  "Bandbreite in mm"
  Massenstrom für Regler/1 -> Massenstrom für Regler Band/1
  Konstante mittlere Dichte/1 -> Massenstrom für Regler/4

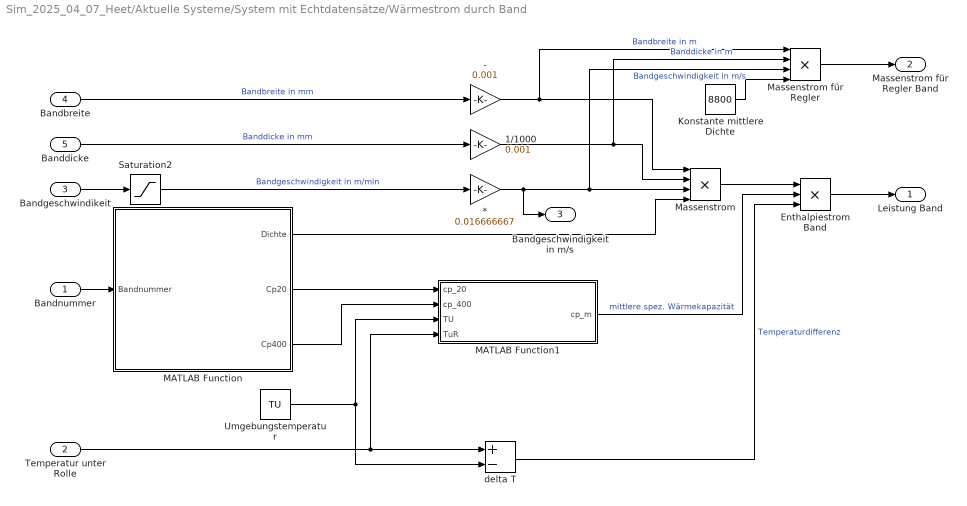
== system Sim_2025_04_07_Heet/Aktuelle Systeme/System mit Echtdatensätze/Wärmestrom durch Band ==
  Bandnummer : Inport
  Temperatur unter Rolle : Inport  Port=2
  Bandgeschwindikeit : Inport  Port=3
  Bandbreite : Inport  Port=4
  Banddicke : Inport  Port=5
  * : Gain  Gain=0.016666667
  - : Gain  Gain=0.001
  1/1000 : Gain  Gain=0.001
  Enthalpiestrom Band : Product  Inputs=3
  Konstante mittlere Dichte : Constant  Value=8800
  MATLAB Function : MATLAB Function  TreatAsAtomicUnit=on
  MATLAB Function1 : MATLAB Function  TreatAsAtomicUnit=on
  Massenstrom : Product  Inputs=4
  Massenstrom für Regler : Product  Inputs=4
  Saturation2 : Saturate  UpperLimit=inf  LowerLimit=0
  Umgebungstemperatur : Constant  Value=TU
  delta T : Sum  Inputs=+-
  Leistung Band : Outport
  Massenstrom für Regler Band : Outport  Port=2
  Bandgeschwindigkeit in m/s : Outport  Port=3
  wires:
  Konstante mittlere Dichte/1 -> Massenstrom für Regler/4
  Massenstrom für Regler/1 -> Massenstrom für Regler Band/1
  Bandbreite/1 -> -/1  "Bandbreite in mm"
  Massenstrom/1 -> Enthalpiestrom Band/1
  Enthalpiestrom Band/1 -> Leistung Band/1
  Saturation2/1 -> */1  "Bandgeschwindigkeit in m/min"
  delta T/1 -> Enthalpiestrom Band/3  "Temperaturdifferenz"
  MATLAB Function/2(Cp20) -> MATLAB Function1/1(cp_20)
  MATLAB Function/3(Cp400) -> MATLAB Function1/2(cp_400)
  Umgebungstemperatur/1 -> delta T/2, MATLAB Function1/3(TU)
  MATLAB Function1/1(cp_m) -> Enthalpiestrom Band/2  "mittlere spez. Wärmekapazität"
  MATLAB Function/1(Dichte) -> Massenstrom/4
  Bandnummer/1 -> MATLAB Function/1(Bandnummer)
  */1 -> Bandgeschwindigkeit in m/s/1, Massenstrom/3, Massenstrom für Regler/3  "Bandgeschwindigkeit in m/s"
  -/1 -> Massenstrom/1, Massenstrom für Regler/1  "Bandbreite in m"
  Banddicke/1 -> 1/1000/1  "Banddicke in mm"
  Bandgeschwindikeit/1 -> Saturation2/1
  Temperatur unter Rolle/1 -> MATLAB Function1/4(TuR), delta T/1
  1/1000/1 -> Massenstrom/2, Massenstrom für Regler/2  "Banddicke in m"

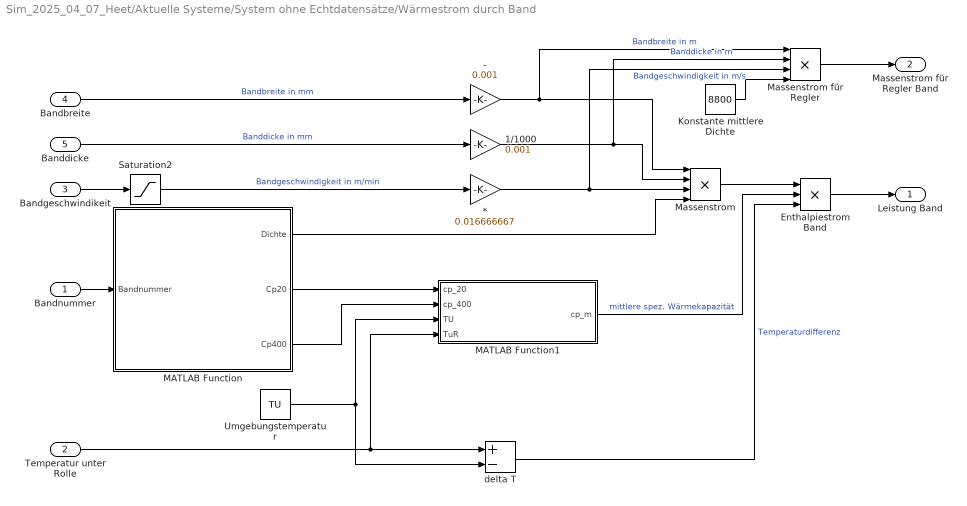
== system Sim_2025_04_07_Heet/Aktuelle Systeme/System ohne Echtdatensätze/Wärmestrom durch Band ==
  Bandnummer : Inport
  Temperatur unter Rolle : Inport  Port=2
  Bandgeschwindikeit : Inport  Port=3
  Bandbreite : Inport  Port=4
  Banddicke : Inport  Port=5
  * : Gain  Gain=0.016666667
  - : Gain  Gain=0.001
  1/1000 : Gain  Gain=0.001
  Enthalpiestrom Band : Product  Inputs=3
  Konstante mittlere Dichte : Constant  Value=8800
  MATLAB Function : MATLAB Function  TreatAsAtomicUnit=on
  MATLAB Function1 : MATLAB Function  TreatAsAtomicUnit=on
  Massenstrom : Product  Inputs=4
  Massenstrom für Regler : Product  Inputs=4
  Saturation2 : Saturate  UpperLimit=inf  LowerLimit=0
  Umgebungstemperatur : Constant  Value=TU
  delta T : Sum  Inputs=+-
  Leistung Band : Outport
  Massenstrom für Regler Band : Outport  Port=2
  wires:
  1/1000/1 -> Massenstrom für Regler/2, Massenstrom/2  "Banddicke in m"
  Temperatur unter Rolle/1 -> delta T/1, MATLAB Function1/4(TuR)
  Bandgeschwindikeit/1 -> Saturation2/1
  Banddicke/1 -> 1/1000/1  "Banddicke in mm"
  -/1 -> Massenstrom für Regler/1, Massenstrom/1  "Bandbreite in m"
  */1 -> Massenstrom für Regler/3, Massenstrom/3  "Bandgeschwindigkeit in m/s"
  Bandnummer/1 -> MATLAB Function/1(Bandnummer)
  MATLAB Function/1(Dichte) -> Massenstrom/4
  MATLAB Function1/1(cp_m) -> Enthalpiestrom Band/2  "mittlere spez. Wärmekapazität"
  Umgebungstemperatur/1 -> MATLAB Function1/3(TU), delta T/2
  MATLAB Function/3(Cp400) -> MATLAB Function1/2(cp_400)
  MATLAB Function/2(Cp20) -> MATLAB Function1/1(cp_20)
  delta T/1 -> Enthalpiestrom Band/3  "Temperaturdifferenz"
  Saturation2/1 -> */1  "Bandgeschwindigkeit in m/min"
  Enthalpiestrom Band/1 -> Leistung Band/1
  Massenstrom/1 -> Enthalpiestrom Band/1
  Bandbreite/1 -> -/1  "Bandbreite in mm"
  Massenstrom für Regler/1 -> Massenstrom für Regler Band/1
  Konstante mittlere Dichte/1 -> Massenstrom für Regler/4

== system Sim_2025_04_07_Heet/Alte Systeme/Subsystem1/Wärmestrom durch Band ==
  Bandnummer : Inport
  Temperatur unter Rolle : Inport  Port=2
  Bandgeschwindikeit : Inport  Port=3
  Bandbreite : Inport  Port=4
  Banddicke : Inport  Port=5
  * : Gain  Gain=0.016666667
  - : Gain  Gain=0.001
  1/1000 : Gain  Gain=0.001
  Enthalpiestrom Band : Product  Inputs=3
  Konstante mittlere Dichte : Constant  Value=8800
  MATLAB Function : MATLAB Function  TreatAsAtomicUnit=on
  MATLAB Function1 : MATLAB Function  TreatAsAtomicUnit=on
  Massenstrom : Product  Inputs=4
  Massenstrom für Regler : Product  Inputs=4
  Saturation2 : Saturate  UpperLimit=inf  LowerLimit=0
  Umgebungstemperatur : Constant  Value=TU
  delta T : Sum  Inputs=+-
  Leistung Band : Outport
  wires:
  Konstante mittlere Dichte/1 -> Massenstrom für Regler/4
  Massenstrom für Regler/1 -> ?
  Bandbreite/1 -> -/1  "Bandbreite in mm"
  Massenstrom/1 -> Enthalpiestrom Band/1
  Enthalpiestrom Band/1 -> Leistung Band/1
  Saturation2/1 -> */1  "Bandgeschwindigkeit in m/min"
  delta T/1 -> Enthalpiestrom Band/3  "Temperaturdifferenz"
  MATLAB Function/2(Cp20) -> MATLAB Function1/1(cp_20)
  MATLAB Function/3(Cp400) -> MATLAB Function1/2(cp_400)
  Umgebungstemperatur/1 -> delta T/2, MATLAB Function1/3(TU)
  MATLAB Function1/1(cp_m) -> Enthalpiestrom Band/2  "mittlere spez. Wärmekapazität"
  MATLAB Function/1(Dichte) -> Massenstrom/4
  Bandnummer/1 -> MATLAB Function/1(Bandnummer)
  */1 -> Massenstrom/3, Massenstrom für Regler/3  "Bandgeschwindigkeit in m/s"
  -/1 -> Massenstrom/1, Massenstrom für Regler/1  "Bandbreite in m"
  Banddicke/1 -> 1/1000/1  "Banddicke in mm"
  Bandgeschwindikeit/1 -> Saturation2/1
  Temperatur unter Rolle/1 -> MATLAB Function1/4(TuR), delta T/1
  1/1000/1 -> Massenstrom/2, Massenstrom für Regler/2  "Banddicke in m"

== system Sim_2025_04_07_Heet/Alte Systeme/Subsystem2/Wärmestrom durch Band ==
  Bandnummer : Inport
  Temperatur unter Rolle : Inport  Port=2
  Bandgeschwindikeit : Inport  Port=3
  Bandbreite : Inport  Port=4
  Banddicke : Inport  Port=5
  * : Gain  Gain=0.016666667
  - : Gain  Gain=0.001
  1/1000 : Gain  Gain=0.001
  Enthalpiestrom Band : Product  Inputs=3
  Konstante mittlere Dichte : Constant  Value=8800
  MATLAB Function : MATLAB Function  TreatAsAtomicUnit=on
  MATLAB Function1 : MATLAB Function  TreatAsAtomicUnit=on
  Massenstrom : Product  Inputs=4
  Massenstrom für Regler : Product  Inputs=4
  Saturation2 : Saturate  UpperLimit=inf  LowerLimit=0
  Umgebungstemperatur : Constant  Value=TU
  delta T : Sum  Inputs=+-
  Leistung Band : Outport
  wires:
  Konstante mittlere Dichte/1 -> Massenstrom für Regler/4
  Massenstrom für Regler/1 -> ?
  Bandbreite/1 -> -/1  "Bandbreite in mm"
  Massenstrom/1 -> Enthalpiestrom Band/1
  Enthalpiestrom Band/1 -> Leistung Band/1
  Saturation2/1 -> */1  "Bandgeschwindigkeit in m/min"
  delta T/1 -> Enthalpiestrom Band/3  "Temperaturdifferenz"
  MATLAB Function/2(Cp20) -> MATLAB Function1/1(cp_20)
  MATLAB Function/3(Cp400) -> MATLAB Function1/2(cp_400)
  Umgebungstemperatur/1 -> delta T/2, MATLAB Function1/3(TU)
  MATLAB Function1/1(cp_m) -> Enthalpiestrom Band/2  "mittlere spez. Wärmekapazität"
  MATLAB Function/1(Dichte) -> Massenstrom/4
  Bandnummer/1 -> MATLAB Function/1(Bandnummer)
  */1 -> Massenstrom/3, Massenstrom für Regler/3  "Bandgeschwindigkeit in m/s"
  -/1 -> Massenstrom/1, Massenstrom für Regler/1  "Bandbreite in m"
  Banddicke/1 -> 1/1000/1  "Banddicke in mm"
  Bandgeschwindikeit/1 -> Saturation2/1
  Temperatur unter Rolle/1 -> MATLAB Function1/4(TuR), delta T/1
  1/1000/1 -> Massenstrom/2, Massenstrom für Regler/2  "Banddicke in m"

== system Sim_2025_04_07_Heet/Alte Systeme/Subsystem3/Wärmestrom durch Band ==
  Bandnummer : Inport
  Temperatur unter Rolle : Inport  Port=2
  Bandgeschwindikeit : Inport  Port=3
  Bandbreite : Inport  Port=4
  Banddicke : Inport  Port=5
  * : Gain  Gain=0.016666667
  - : Gain  Gain=0.001
  1/1000 : Gain  Gain=0.001
  Enthalpiestrom Band : Product  Inputs=3
  Konstante mittlere Dichte : Constant  Value=8800
  MATLAB Function : MATLAB Function  TreatAsAtomicUnit=on
  MATLAB Function1 : MATLAB Function  TreatAsAtomicUnit=on
  Massenstrom : Product  Inputs=4
  Massenstrom für Regler : Product  Inputs=4
  Saturation2 : Saturate  UpperLimit=inf  LowerLimit=0
  Umgebungstemperatur : Constant  Value=TU
  delta T : Sum  Inputs=+-
  Leistung Band : Outport
  Massenstrom für Regler Band : Outport  Port=2
  wires:
  Konstante mittlere Dichte/1 -> Massenstrom für Regler/4
  Massenstrom für Regler/1 -> Massenstrom für Regler Band/1
  Bandbreite/1 -> -/1  "Bandbreite in mm"
  Massenstrom/1 -> Enthalpiestrom Band/1
  Enthalpiestrom Band/1 -> Leistung Band/1
  Saturation2/1 -> */1  "Bandgeschwindigkeit in m/min"
  delta T/1 -> Enthalpiestrom Band/3  "Temperaturdifferenz"
  MATLAB Function/2(Cp20) -> MATLAB Function1/1(cp_20)
  MATLAB Function/3(Cp400) -> MATLAB Function1/2(cp_400)
  Umgebungstemperatur/1 -> delta T/2, MATLAB Function1/3(TU)
  MATLAB Function1/1(cp_m) -> Enthalpiestrom Band/2  "mittlere spez. Wärmekapazität"
  MATLAB Function/1(Dichte) -> Massenstrom/4
  Bandnummer/1 -> MATLAB Function/1(Bandnummer)
  */1 -> Massenstrom/3, Massenstrom für Regler/3  "Bandgeschwindigkeit in m/s"
  -/1 -> Massenstrom/1, Massenstrom für Regler/1  "Bandbreite in m"
  Banddicke/1 -> 1/1000/1  "Banddicke in mm"
  Bandgeschwindikeit/1 -> Saturation2/1
  Temperatur unter Rolle/1 -> MATLAB Function1/4(TuR), delta T/1
  1/1000/1 -> Massenstrom/2, Massenstrom für Regler/2  "Banddicke in m"

== system Sim_2025_04_07_Heet/Alte Systeme/Subsystem4/Wärmestrom durch Band ==
  Bandnummer : Inport
  Temperatur unter Rolle : Inport  Port=2
  Bandgeschwindikeit : Inport  Port=3
  Bandbreite : Inport  Port=4
  Banddicke : Inport  Port=5
  * : Gain  Gain=0.016666667
  - : Gain  Gain=0.001
  1/1000 : Gain  Gain=0.001
  Enthalpiestrom Band : Product  Inputs=3
  Konstante mittlere Dichte : Constant  Value=8800
  MATLAB Function : MATLAB Function  TreatAsAtomicUnit=on
  MATLAB Function1 : MATLAB Function  TreatAsAtomicUnit=on
  Massenstrom : Product  Inputs=4
  Massenstrom für Regler : Product  Inputs=4
  Saturation2 : Saturate  UpperLimit=inf  LowerLimit=0
  Umgebungstemperatur : Constant  Value=TU
  delta T : Sum  Inputs=+-
  Leistung Band : Outport
  Massenstrom für Regler Band : Outport  Port=2
  wires:
  Konstante mittlere Dichte/1 -> Massenstrom für Regler/4
  Massenstrom für Regler/1 -> Massenstrom für Regler Band/1
  Bandbreite/1 -> -/1  "Bandbreite in mm"
  Massenstrom/1 -> Enthalpiestrom Band/1
  Enthalpiestrom Band/1 -> Leistung Band/1
  Saturation2/1 -> */1  "Bandgeschwindigkeit in m/min"
  delta T/1 -> Enthalpiestrom Band/3  "Temperaturdifferenz"
  MATLAB Function/2(Cp20) -> MATLAB Function1/1(cp_20)
  MATLAB Function/3(Cp400) -> MATLAB Function1/2(cp_400)
  Umgebungstemperatur/1 -> delta T/2, MATLAB Function1/3(TU)
  MATLAB Function1/1(cp_m) -> Enthalpiestrom Band/2  "mittlere spez. Wärmekapazität"
  MATLAB Function/1(Dichte) -> Massenstrom/4
  Bandnummer/1 -> MATLAB Function/1(Bandnummer)
  */1 -> Massenstrom/3, Massenstrom für Regler/3  "Bandgeschwindigkeit in m/s"
  -/1 -> Massenstrom/1, Massenstrom für Regler/1  "Bandbreite in m"
  Banddicke/1 -> 1/1000/1  "Banddicke in mm"
  Bandgeschwindikeit/1 -> Saturation2/1
  Temperatur unter Rolle/1 -> MATLAB Function1/4(TuR), delta T/1
  1/1000/1 -> Massenstrom/2, Massenstrom für Regler/2  "Banddicke in m"

== matlab function Sim_2025_04_07_Heet/Alte Systeme/Subsystem2/Air knife Betriebszustandsberechnung in Prozent ==
  data: druck1 input; druck2 input; Prozent output
function Prozent  = fcn(druck1, druck2)
%#codegen
% fcn Berechnet die Leistung und den prozentualen Anteil mithilfe einer
%     natürlichen Logarithmusfunktion.
%
% Eingänge:
%   druck1 - Erster Druckwert in mbar
%   druck2 - Zweiter Druckwert in mbar
%
% Ausgänge:
%   Leistung - Berechnete Leistung in Watt
%   Prozent  - Relativer Anteil in Prozent (0% - 100%)
%
% Randbedingungen:
%   - 0 mbar => 0%
%   - 400 mbar => 100%
%   - Dazwischen natürliche Logarithmus-Skalierung

    % Mittelwert berechnen
    druckMittelwert = (druck1 + druck2) / 2;
    
    % Sicherheitsabfragen, um log(0) zu vermeiden
    if druckMittelwert < 20
        druckMittelwert = 0;
    elseif druckMittelwert > 600
        druckMittelwert = 600;
    end

    
    if druckMittelwert == 0
        Prozent = 0;
    else
        Prozent = 100 *druckMittelwert / 600;
    end

    Leistung = (Prozent / 100) * 25900;
end

== matlab function Sim_2025_04_07_Heet/Alte Systeme/Subsystem2/Wärmestrom durch Band/MATLAB Function ==
  data: Bandnummer input; Dichte output; Cp20 output; Cp400 output
function [Dichte, Cp20, Cp400] = materialdaten(Bandnummer)
    % Materialdaten Tabelle
    Nr = (1:18)';

    % Dichte in kg/m³ (Umrechnung von g/cm³: * 1000)
    DichteList = [8960; 8960; 8900; 8850; 8800; 8800; 8800; 8800; 8750; 8750; 8900; 8900; 8900; 8800; 8800; 8900; 8900; 8200];

    % Thermische Leitfähigkeit bei 20°C in W/(m K)
    T_Leitfaeh20CList = [385; 385; 84; 82; 75; 75; 62; 62; 50; 120; 300; 260; 245; 190; 161; 197; 161; 81];

    % Thermische Leitfähigkeit bei 270°C in W/(m K)
    T_Leitfaeh270CList = [375; 375; 67; 35; 60; 60; 49; 49; 40; 103; 288; 214; 207; 160; 140; 175; 140; 68];

    % Wärmeausdehnungskoeffizient β in 1/K
    WaermeausdehnungskoefList = [1.77E-05; 1.77E-05; 1.82E-05; 1.82E-05; 1.85E-05; 1.85E-05; 1.85E-05; 1.85E-05; 1.84E-05; 1.84E-05; 1.80E-05; 1.68E-05; 1.68E-05; 1.70E-05; 1.70E-05; 1.70E-05; 1.70E-05; 1.82E-05];

    % Spezifische Wärmekapazität cp in J/(kg K) bei 20°C, 200°C, 400°C
    Cp20List = [385; 385; 360; 350; 340; 340; 330; 325; 320; 330; 385; 380; 375; 360; 365; 360; 355; 350];

    Cp200List = [388; 388; 370; 360; 360; 360; 340; 335; 340; 340; 388; 385; 380; 370; 375; 370; 365; 360];

    Cp400List = [391; 391; 380; 370; 370; 370; 350; 345; 350; 350; 391; 390; 385; 380; 380; 375; 370; 370];
    
    % Initialisierung der Ausgänge
    Dichte = 0;
    T_Leitfaeh20C = 0;
    T_Leitfaeh270C = 0;
    Waermeausdehnungskoef = 0;
    Cp20 = 0;
    Cp200 = 0;
    Cp400 = 0;

    % Prüfen, ob die Bandnummer gültig ist
    if Bandnummer > 0 && Bandnummer <= length(Nr)
        Dichte = DichteList(Bandnummer);
        T_Leitfaeh20C = T_Leitfaeh20CList(Bandnummer);
        T_Leitfaeh270C = T_Leitfaeh270CList(Bandnummer);
        Waermeausdehnungskoef = WaermeausdehnungskoefList(Bandnummer);
        Cp20 = Cp20List(Bandnummer);
        Cp200 = Cp200List(Bandnummer);
        Cp400 = Cp400List(Bandnummer);
    end
end

== matlab function Sim_2025_04_07_Heet/Alte Systeme/Subsystem2/Wärmestrom durch Band/MATLAB Function1 ==
  data: cp_20 input; cp_m output; cp_400 input; TU input; TuR input
function cp_m = cp_abhaengig_T(cp_20, cp_400, TU, TuR)
% Funktion zur Berechnung der Wärmekapazität bei der mittleren Temperatur

    % Mittlere Temperatur berechnen
    Tm = (TU + TuR) / 2;

    % Lineare Interpolation der Wärmekapazität
    % Annahme: Wärmekapazität ändert sich linear zwischen 20°C und 400°C
    cp_m = cp_20 + (cp_400 - cp_20) * (Tm - 20) / (400 - 20);

end
